simulink model "simulation"  (R2018a)
settings: Solver=VariableStepAuto  StartTime=0.0  StopTime=251/1004+1/192000  RelTol=1e-3
libraries: dspspect3 x1, dspsrcs4 x1
settings Model: Creator=Christopher  LastModifiedBy=Christopher

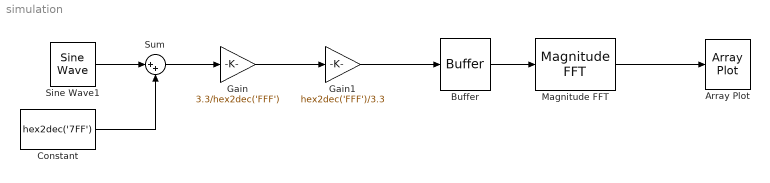
== system simulation ==
  Array Plot : ArrayPlot
  Buffer : Buffer  N=4096  OutputFrames=off
  Constant : Constant  Value=hex2dec('7FF')
  Gain : Gain  Gain=3.3/hex2dec('FFF')
  Gain1 : Gain  Gain=hex2dec('FFF')/3.3
  Magnitude FFT : dspspect3/Magnitude FFT  mag_or_magsq=Magnitude squared  FFTImplementation=Auto  fftLenInherit=off  fftsize=4096  WrapInput=on
      settings: SourceProductName=DSP System Toolbox  SourceProductBaseCode=DS
  Sine Wave1 : dspsrcs4/Sine Wave  Amplitude=hex2dec('7FF')  Frequency=1004  Phase=0  SampleMode=Discrete  OutComplex=Real  CompMethod=Trigonometric fcn  TableSize=Speed  SampleTime=1/192000  SamplesPerFrame=1  ResetState=Restart at time zero  OutputFrames=off  dataType=double  wordLen=16  udDataType=sfix(16)  fracBitsMode=Best precision  numFracBits=15  OutDataTypeStr=double  LastOutDataTypeStr=double
  Sum : Sum  Inputs=|++
  wires:
  Sine Wave1/1 -> Sum/1
  Constant/1 -> Sum/2
  Sum/1 -> Gain/1
  Gain/1 -> Gain1/1
  Magnitude FFT/1 -> Array Plot/1
  Gain1/1 -> Buffer/1
  Buffer/1 -> Magnitude FFT/1
